simulink model "lots_of_connections"  (Simulink 7.6)
settings: Solver=FixedStepDiscrete  StartTime=0.0  StopTime=0  RelTol=1e-3
values from neighbouring files (symbols this model uses):
  Iter_Segment_Thresh = 60    [VisionConstants.m]
  Scale_Forward_B = 0    [VisionConstants.m]
  Scale_Forward_G = 1    [VisionConstants.m]
  Scale_Forward_H = 1    [VisionConstants.m]
  Scale_Forward_R = 0    [VisionConstants.m]
  Scale_Forward_S = 1    [VisionConstants.m]
  Scale_Forward_V = 5    [VisionConstants.m]
undefined symbols (not defined in the file or in its folder): black_al, black_au, black_bl, black_bu, blue_al, blue_au, blue_bl, blue_bu, gray, green_al, green_au, green_bl, green_bu, orange_al, orange_au, orange_bl, orange_bu, Rec, red_al, red_au, red_bl, red_bu, SDTV, yellow_al, yellow_au, yellow_bl, yellow_bu
libraries: vipconversions x4, vipgeotforms x3, vipsnks x2, vipsrcs x1
settings Model: Creator=Thing 1  LastModifiedBy=auvt
settings OptimizationCC: InlineParams=on  OptimizeModelRefInitCode=on
settings RTWCC: SystemTargetFile=ert.tlc  GenCodeOnly=on  TemplateMakefile=ert_default_tmf  Description=Real-Time Workshop Embedded Coder  GenerateReport=on  ProcessScript=ert_make_rtw_hook  IncludeHyperlinkInReport=on  LaunchReport=on  TargetLang=C++
settings CodeAppCC: IgnoreCustomStorageClasses=off
settings ERTTargetCC: MultiwordLength=2048  GenerateSampleERTMain=on  IncludeMdlTerminateFcn=off  ERTCustomFileTemplate=example_file_process.tlc  ConvertIfToSwitch=off

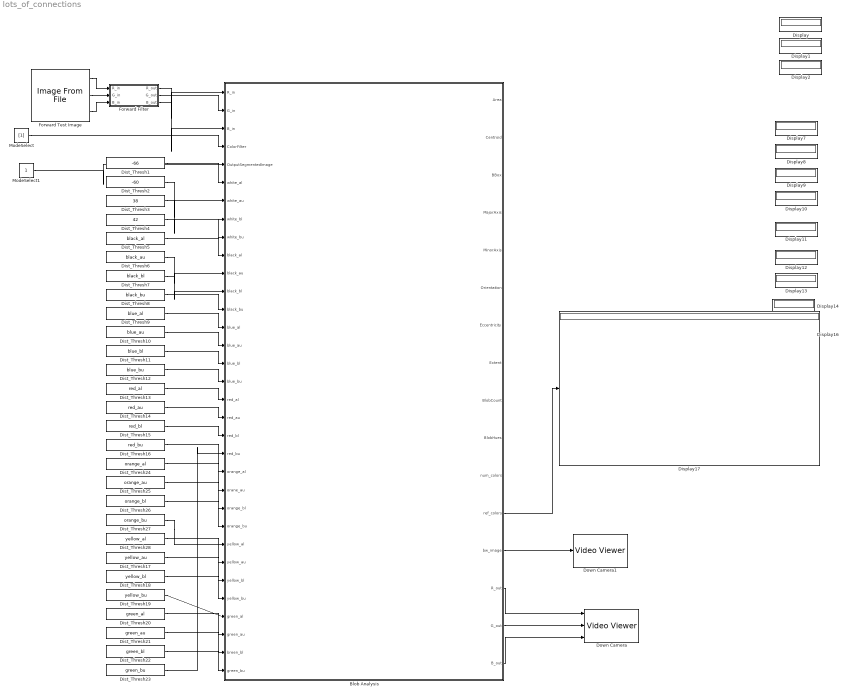
== system lots_of_connections ==
  Blob Analysis : Subsystem
  Display{,1..2,7..14,16..17} (13 alike) : Display
  Dist_Thresh1 : Constant  Value=-66  SampleTime=-1
  Dist_Thresh10 : Constant  Value=blue_au  SampleTime=-1
  Dist_Thresh11 : Constant  Value=blue_bl  SampleTime=-1
  Dist_Thresh12 : Constant  Value=blue_bu  SampleTime=-1
  Dist_Thresh13 : Constant  Value=red_al  SampleTime=-1
  Dist_Thresh14 : Constant  Value=red_au  SampleTime=-1
  Dist_Thresh15 : Constant  Value=red_bl  SampleTime=-1
  Dist_Thresh16 : Constant  Value=red_bu  SampleTime=-1
  Dist_Thresh17 : Constant  Value=yellow_au  SampleTime=-1
  Dist_Thresh18 : Constant  Value=yellow_bl  SampleTime=-1
  Dist_Thresh19 : Constant  Value=yellow_bu  SampleTime=-1
  Dist_Thresh2 : Constant  Value=-60  SampleTime=-1
  Dist_Thresh20 : Constant  Value=green_al  SampleTime=-1
  Dist_Thresh21 : Constant  Value=green_au  SampleTime=-1
  Dist_Thresh22 : Constant  Value=green_bl  SampleTime=-1
  Dist_Thresh23 : Constant  Value=green_bu  SampleTime=-1
  Dist_Thresh24 : Constant  Value=orange_al  SampleTime=-1
  Dist_Thresh25 : Constant  Value=orange_au  SampleTime=-1
  Dist_Thresh26 : Constant  Value=orange_bl  SampleTime=-1
  Dist_Thresh27 : Constant  Value=orange_bu  SampleTime=-1
  Dist_Thresh28 : Constant  Value=yellow_al  SampleTime=-1
  Dist_Thresh3 : Constant  Value=38  SampleTime=-1
  Dist_Thresh4 : Constant  Value=42  SampleTime=-1
  Dist_Thresh5 : Constant  Value=black_al  SampleTime=-1
  Dist_Thresh6 : Constant  Value=black_au  SampleTime=-1
  Dist_Thresh7 : Constant  Value=black_bl  SampleTime=-1
  Dist_Thresh8 : Constant  Value=black_bu  SampleTime=-1
  Dist_Thresh9 : Constant  Value=blue_al  SampleTime=-1
  Down Camera : vipsnks/Video Viewer  DialogControllerArgs=DataTag4  inputType=Obsolete7b  imagePorts=Separate color signals  useColorMap=off  colormapValue=gray(256)  specRange=off  minInputVal=0  maxInputVal=255  FigPos=[565 773 364 553]  AxisZoom=on  trueSizedOnce=off  OpenAtMdlStart=on
  Down Camera1 : vipsnks/Video Viewer  DialogControllerArgs=DataTag6  inputType=Obsolete7b  imagePorts=One multidimensional signal  useColorMap=off  colormapValue=gray(256)  specRange=off  minInputVal=0  maxInputVal=255  FigPos=[955 767 364 553]  AxisZoom=on  trueSizedOnce=off  OpenAtMdlStart=on
  Forward Filter : Subsystem
  Forward Test Image : vipsrcs/Image From File  Tag=vipblks_nd  DialogController=vipDDGCreate  DialogControllerArgs=DataTag7  SystemSampleTime=-1  FileName=/home/auvt/auvc/src/vision/Test_Images/gate10.bmp  imagePorts=Separate color signals  Ts=-1  ImageDataType=double  Signed=on  WordLength=16  sdImageDataType=uint(8)  FractionLengthMode=User-defined  FractionLength=15  OutPortLabels=R|G|B
  ModeSelect : Constant  Value=[1]  SampleTime=-1
  ModeSelect1 : Constant  SampleTime=-1
  wires:
  Dist_Thresh1/1 -> Blob Analysis/6(white_al)
  Dist_Thresh2/1 -> Blob Analysis/7(white_au)
  Dist_Thresh3/1 -> Blob Analysis/8(white_bl)
  Dist_Thresh4/1 -> Blob Analysis/9(white_bu)
  Dist_Thresh5/1 -> Blob Analysis/10(black_al)
  Dist_Thresh6/1 -> Blob Analysis/11(black_au)
  Dist_Thresh7/1 -> Blob Analysis/12(black_bl)
  Dist_Thresh8/1 -> Blob Analysis/13(black_bu)
  Dist_Thresh9/1 -> Blob Analysis/14(blue_al)
  Dist_Thresh10/1 -> Blob Analysis/15(blue_au)
  Dist_Thresh11/1 -> Blob Analysis/16(blue_bl)
  Dist_Thresh12/1 -> Blob Analysis/17(blue_bu)
  Dist_Thresh13/1 -> Blob Analysis/18(red_al)
  Dist_Thresh14/1 -> Blob Analysis/19(red_au)
  Dist_Thresh15/1 -> Blob Analysis/20(red_bl)
  Dist_Thresh16/1 -> Blob Analysis/22(orange_al)
  Dist_Thresh24/1 -> Blob Analysis/23(orane_au)
  Dist_Thresh25/1 -> Blob Analysis/24(orange_bl)
  Dist_Thresh26/1 -> Blob Analysis/25(orange_bu)
  Dist_Thresh27/1 -> Blob Analysis/26(yellow_al)
  Dist_Thresh28/1 -> Blob Analysis/27(yellow_au)
  Dist_Thresh17/1 -> Blob Analysis/28(yellow_bl)
  Dist_Thresh18/1 -> Blob Analysis/29(yellow_bu)
  Dist_Thresh19/1 -> Blob Analysis/30(green_al)
  Dist_Thresh20/1 -> Blob Analysis/31(green_au)
  Dist_Thresh21/1 -> Blob Analysis/32(breen_bl)
  Dist_Thresh22/1 -> Blob Analysis/33(green_bu)
  Dist_Thresh23/1 -> Blob Analysis/21(red_bu)
  Blob Analysis/14(R_out) -> Down Camera/1
  Blob Analysis/15(G_out) -> Down Camera/2
  Blob Analysis/16(B_out) -> Down Camera/3
  ModeSelect/1 -> Blob Analysis/4(ColorFilter)
  ModeSelect1/1 -> Blob Analysis/5(OutputSegmentedImage)
  Blob Analysis/13(bw_image) -> Down Camera1/1
  Blob Analysis/12(ref_colors) -> Display17/1
  Forward Test Image/1 -> Forward Filter/1(R_in)
  Forward Test Image/2 -> Forward Filter/2(G_in)
  Forward Test Image/3 -> Forward Filter/3(B_in)
  Forward Filter/1(R_out) -> Blob Analysis/1(R_in)
  Forward Filter/2(G_out) -> Blob Analysis/2(G_in)
  Forward Filter/3(B_out) -> Blob Analysis/3(B_in)

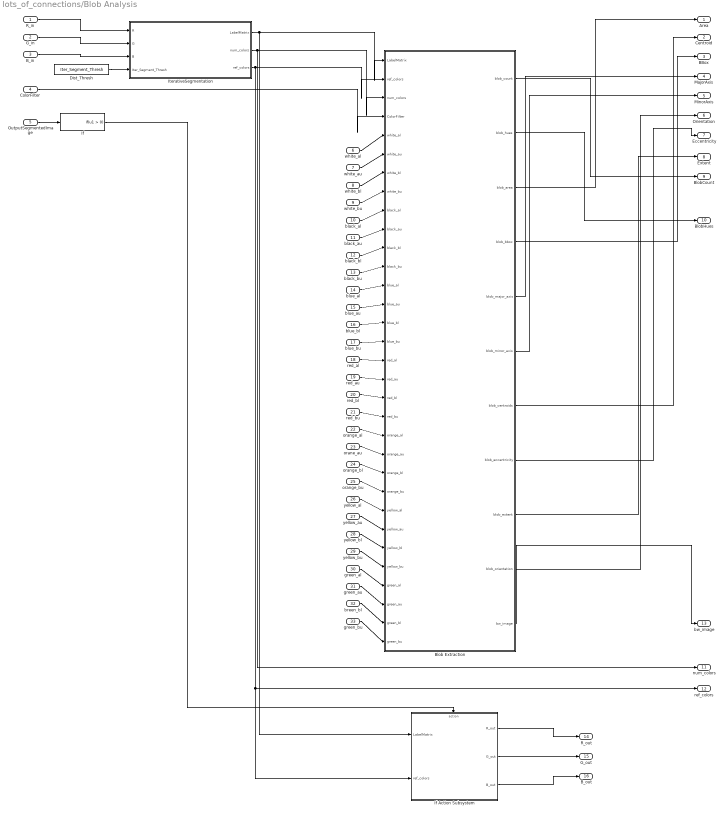
== system lots_of_connections/Blob Analysis ==
  R_in : Inport
  G_in : Inport  Port=2
  B_in : Inport  Port=3
  ColorFilter : Inport  Port=4
  OutputSegmentedImage : Inport  Port=5
  white_al : Inport  Port=6
  white_au : Inport  Port=7
  white_bl : Inport  Port=8
  white_bu : Inport  Port=9
  black_al : Inport  Port=10
  black_au : Inport  Port=11
  black_bl : Inport  Port=12
  black_bu : Inport  Port=13
  blue_al : Inport  Port=14
  blue_au : Inport  Port=15
  blue_bl : Inport  Port=16
  blue_bu : Inport  Port=17
  red_al : Inport  Port=18
  red_au : Inport  Port=19
  red_bl : Inport  Port=20
  red_bu : Inport  Port=21
  orange_al : Inport  Port=22
  orane_au : Inport  Port=23
  orange_bl : Inport  Port=24
  orange_bu : Inport  Port=25
  yellow_al : Inport  Port=26
  yellow_au : Inport  Port=27
  yellow_bl : Inport  Port=28
  yellow_bu : Inport  Port=29
  green_al : Inport  Port=30
  green_au : Inport  Port=31
  breen_bl : Inport  Port=32
  green_bu : Inport  Port=33
  Blob Extraction : Stateflow chart  TreatAsAtomicUnit=on
  Dist_Thresh : Constant  Value=Iter_Segment_Thresh  SampleTime=-1
  If : If  ShowElse=off
  If Action Subsystem : Subsystem  TreatAsAtomicUnit=on
  IterativeSegmentation : Subsystem
      settings: UndoDeleteFcn=Stateflow.SLINSF.SimulinkMan.restorePreDeleteFcn  PreDeleteFcn=Stateflow.SLINSF.SimulinkMan.removePreDeleteFcn
  Area : Outport
  Centroid : Outport  Port=2
  BBox : Outport  Port=3
  MajorAxis : Outport  Port=4
  MinorAxis : Outport  Port=5
  Orientation : Outport  Port=6
  Eccentricity : Outport  Port=7
  Extent : Outport  Port=8
  BlobCount : Outport  Port=9
  BlobHues : Outport  Port=10
  num_colors : Outport  Port=11
  ref_colors : Outport  Port=12
  bw_image : Outport  Port=13
  R_out : Outport  Port=14
  G_out : Outport  Port=15
  B_out : Outport  Port=16
  wires:
  IterativeSegmentation/1(LabelMatrix) -> Blob Extraction/1(LabelMatrix), If Action Subsystem/1(LabelMatrix)
  IterativeSegmentation/2(num_colors) -> Blob Extraction/3(num_colors), num_colors/1
  IterativeSegmentation/3(ref_colors) -> Blob Extraction/2(ref_colors), If Action Subsystem/2(ref_colors), ref_colors/1
  Blob Extraction/3(blob_area) -> Area/1
  Blob Extraction/7(blob_centroids) -> Centroid/1
  Blob Extraction/4(blob_bbox) -> BBox/1
  Blob Extraction/5(blob_major_axis) -> MajorAxis/1
  Blob Extraction/6(blob_minor_axis) -> MinorAxis/1
  Blob Extraction/10(blob_orientation) -> Orientation/1
  Blob Extraction/8(blob_eccentricity) -> Eccentricity/1
  Blob Extraction/9(blob_extent) -> Extent/1
  Blob Extraction/1(blob_count) -> BlobCount/1
  Blob Extraction/2(blob_hues) -> BlobHues/1
  ColorFilter/1 -> Blob Extraction/4(ColorFilter)
  Dist_Thresh/1 -> IterativeSegmentation/4(Iter_Segment_Thresh)
  R_in/1 -> IterativeSegmentation/1(R)
  G_in/1 -> IterativeSegmentation/2(G)
  B_in/1 -> IterativeSegmentation/3(B)
  white_al/1 -> Blob Extraction/5(white_al)
  white_au/1 -> Blob Extraction/6(white_au)
  white_bl/1 -> Blob Extraction/7(white_bl)
  white_bu/1 -> Blob Extraction/8(white_bu)
  black_al/1 -> Blob Extraction/9(black_al)
  black_au/1 -> Blob Extraction/10(black_au)
  black_bl/1 -> Blob Extraction/11(black_bl)
  black_bu/1 -> Blob Extraction/12(black_bu)
  blue_al/1 -> Blob Extraction/13(blue_al)
  blue_au/1 -> Blob Extraction/14(blue_au)
  blue_bl/1 -> Blob Extraction/15(blue_bl)
  blue_bu/1 -> Blob Extraction/16(blue_bu)
  red_al/1 -> Blob Extraction/17(red_al)
  red_au/1 -> Blob Extraction/18(red_au)
  red_bl/1 -> Blob Extraction/19(red_bl)
  red_bu/1 -> Blob Extraction/20(red_bu)
  orange_al/1 -> Blob Extraction/21(orange_al)
  orane_au/1 -> Blob Extraction/22(orange_au)
  orange_bl/1 -> Blob Extraction/23(orange_bl)
  orange_bu/1 -> Blob Extraction/24(orange_bu)
  yellow_al/1 -> Blob Extraction/25(yellow_al)
  yellow_au/1 -> Blob Extraction/26(yellow_au)
  yellow_bl/1 -> Blob Extraction/27(yellow_bl)
  yellow_bu/1 -> Blob Extraction/28(yellow_bu)
  green_al/1 -> Blob Extraction/29(green_al)
  green_au/1 -> Blob Extraction/30(green_au)
  breen_bl/1 -> Blob Extraction/31(green_bl)
  green_bu/1 -> Blob Extraction/32(green_bu)
  If/1 -> If Action Subsystem/Action
  OutputSegmentedImage/1 -> If/1
  If Action Subsystem/1(R_out) -> R_out/1
  If Action Subsystem/2(G_out) -> G_out/1
  If Action Subsystem/3(B_out) -> B_out/1
  Blob Extraction/11(bw_image) -> bw_image/1

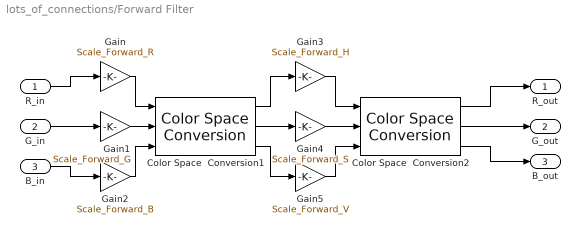
== system lots_of_connections/Forward Filter ==
  R_in : Inport  PortDimensions=Forward_Camera_Dimensions
  G_in : Inport  Port=2  PortDimensions=Forward_Camera_Dimensions
  B_in : Inport  Port=3  PortDimensions=Forward_Camera_Dimensions
  Color Space  Conversion1 : vipconversions/Color Space  Conversion  conversion=Obsolete  conversionActive=R'G'B' to HSV  wp_str=D50  rec=Rec. 601 (SDTV)  sys=1125/60/2:1  imagePorts=Separate color signals
  Color Space  Conversion2 : vipconversions/Color Space  Conversion  conversion=Obsolete  conversionActive=HSV to R'G'B'  wp_str=D50  rec=Rec. 601 (SDTV)  sys=1125/60/2:1  imagePorts=Separate color signals
  Gain : Gain  Gain=Scale_Forward_R
  Gain1 : Gain  Gain=Scale_Forward_G
  Gain2 : Gain  Gain=Scale_Forward_B
  Gain3 : Gain  Gain=Scale_Forward_H
  Gain4 : Gain  Gain=Scale_Forward_S
  Gain5 : Gain  Gain=Scale_Forward_V
  R_out : Outport  OutDataTypeStr=double
  G_out : Outport  Port=2  OutDataTypeStr=double
  B_out : Outport  Port=3  OutDataTypeStr=double
  wires:
  R_in/1 -> Gain/1
  G_in/1 -> Gain1/1
  B_in/1 -> Gain2/1
  Gain/1 -> Color Space  Conversion1/1
  Gain1/1 -> Color Space  Conversion1/2
  Gain2/1 -> Color Space  Conversion1/3
  Color Space  Conversion1/1 -> Gain3/1
  Color Space  Conversion1/2 -> Gain4/1
  Color Space  Conversion1/3 -> Gain5/1
  Gain3/1 -> Color Space  Conversion2/1
  Gain4/1 -> Color Space  Conversion2/2
  Gain5/1 -> Color Space  Conversion2/3
  Color Space  Conversion2/1 -> R_out/1
  Color Space  Conversion2/2 -> G_out/1
  Color Space  Conversion2/3 -> B_out/1

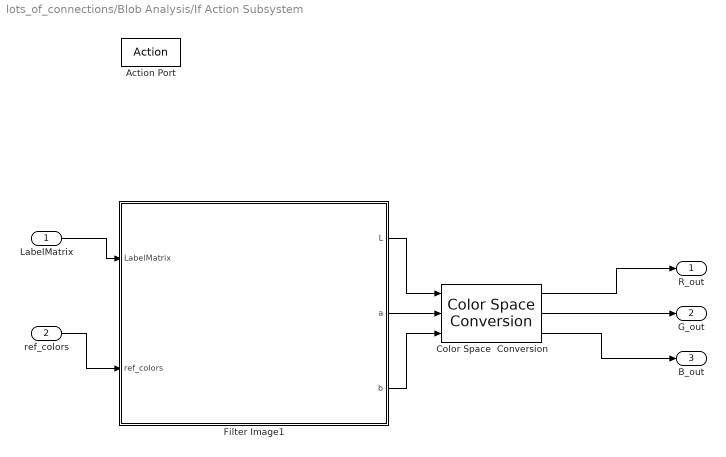
== system lots_of_connections/Blob Analysis/If Action Subsystem ==
  LabelMatrix : Inport
  ref_colors : Inport  Port=2
  Action Port : ActionPort  ActionType=then
  Color Space  Conversion : vipconversions/Color Space  Conversion  conversion=Obsolete  conversionActive=L*a*b* to sR'G'B'  wp_str=D65  rec=Rec. 601 (SDTV)  sys=1125/60/2:1  imagePorts=Separate color signals
  Filter Image1 : Stateflow chart  TreatAsAtomicUnit=on
  R_out : Outport
  G_out : Outport  Port=2
  B_out : Outport  Port=3
  wires:
  LabelMatrix/1 -> Filter Image1/1(LabelMatrix)
  ref_colors/1 -> Filter Image1/2(ref_colors)
  Filter Image1/1(L) -> Color Space  Conversion/1
  Filter Image1/2(a) -> Color Space  Conversion/2
  Filter Image1/3(b) -> Color Space  Conversion/3
  Color Space  Conversion/1 -> R_out/1
  Color Space  Conversion/2 -> G_out/1
  Color Space  Conversion/3 -> B_out/1

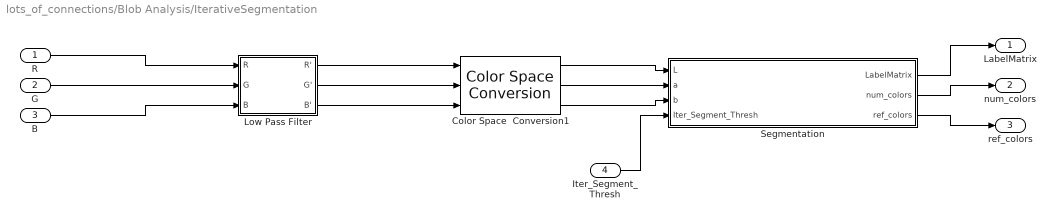
== system lots_of_connections/Blob Analysis/IterativeSegmentation ==
  R : Inport
  G : Inport  Port=2
  B : Inport  Port=3
  Iter_Segment_Thresh : Inport  Port=4
  Color Space  Conversion1 : vipconversions/Color Space  Conversion  conversion=Obsolete  conversionActive=sR'G'B' to L*a*b*  wp_str=D50  rec=Rec. 601 (SDTV)  sys=1125/60/2:1  imagePorts=Separate color signals
  Low Pass Filter : Subsystem
  Segmentation : Subsystem
  LabelMatrix : Outport
  num_colors : Outport  Port=2
  ref_colors : Outport  Port=3
  wires:
  Low Pass Filter/3(B') -> Color Space  Conversion1/3
  Low Pass Filter/2(G') -> Color Space  Conversion1/2
  Low Pass Filter/1(R') -> Color Space  Conversion1/1
  Color Space  Conversion1/3 -> Segmentation/3(b)
  Color Space  Conversion1/2 -> Segmentation/2(a)
  Color Space  Conversion1/1 -> Segmentation/1(L)
  R/1 -> Low Pass Filter/1(R)
  G/1 -> Low Pass Filter/2(G)
  B/1 -> Low Pass Filter/3(B)
  Segmentation/1(LabelMatrix) -> LabelMatrix/1
  Segmentation/2(num_colors) -> num_colors/1
  Segmentation/3(ref_colors) -> ref_colors/1
  Iter_Segment_Thresh/1 -> Segmentation/4(Iter_Segment_Thresh)

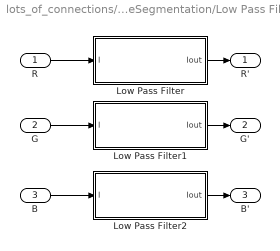
== system lots_of_connections/Blob Analysis/IterativeSegmentation/Low Pass Filter ==
  R : Inport
  G : Inport  Port=2
  B : Inport  Port=3
  Low Pass Filter : Stateflow chart  TreatAsAtomicUnit=on
  Low Pass Filter1 : Stateflow chart  TreatAsAtomicUnit=on
  Low Pass Filter2 : Stateflow chart  TreatAsAtomicUnit=on
  R' : Outport
  G' : Outport  Port=2
  B' : Outport  Port=3
  wires:
  Low Pass Filter/1(Iout) -> R'/1
  Low Pass Filter2/1(Iout) -> B'/1
  Low Pass Filter1/1(Iout) -> G'/1
  B/1 -> Low Pass Filter2/1(I)
  G/1 -> Low Pass Filter1/1(I)
  R/1 -> Low Pass Filter/1(I)

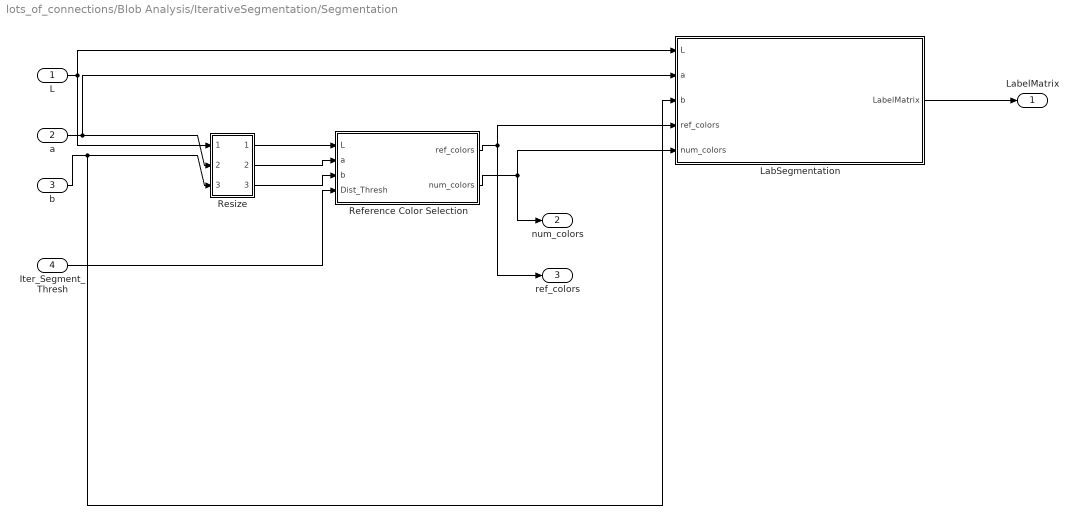
== system lots_of_connections/Blob Analysis/IterativeSegmentation/Segmentation ==
  L : Inport
  a : Inport  Port=2
  b : Inport  Port=3
  Iter_Segment_Thresh : Inport  Port=4
  LabSegmentation : Stateflow chart  TreatAsAtomicUnit=on
  Reference Color Selection : Stateflow chart  TreatAsAtomicUnit=on
  Resize : Subsystem
  LabelMatrix : Outport
  num_colors : Outport  Port=2
  ref_colors : Outport  Port=3
  wires:
  Iter_Segment_Thresh/1 -> Reference Color Selection/4(Dist_Thresh)
  LabSegmentation/1(LabelMatrix) -> LabelMatrix/1
  Reference Color Selection/2(num_colors) -> LabSegmentation/5(num_colors), num_colors/1
  Reference Color Selection/1(ref_colors) -> ref_colors/1, LabSegmentation/4(ref_colors)
  Resize/3(Out3) -> Reference Color Selection/3(b)
  Resize/2(Out2) -> Reference Color Selection/2(a)
  Resize/1(Out1) -> Reference Color Selection/1(L)
  b/1 -> LabSegmentation/3(b), Resize/3(In3)
  a/1 -> LabSegmentation/2(a), Resize/2(In2)
  L/1 -> LabSegmentation/1(L), Resize/1(In1)

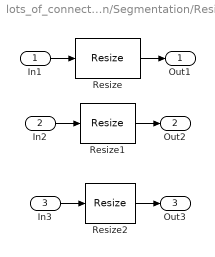
== system lots_of_connections/Blob Analysis/IterativeSegmentation/Segmentation/Resize ==
  In1 : Inport
  In2 : Inport  Port=2
  In3 : Inport  Port=3
  Resize : vipgeotforms/Resize  DialogController=vipDDGCreate  DialogControllerArgs=DataTag0  specify=Number of output rows and columns  rfactor=[]  outCols=25  outRows=25  outRowsCols=[60 80]  interp_method=Bilinear  antialias=on  useROI=off  roiFlag=off  prodOutputMode=Binary point scaling  prodOutputWordLength=32  prodOutputFracLength=10  roundingMode=Nearest  overflowMode=on
  Resize1 : vipgeotforms/Resize  DialogController=vipDDGCreate  DialogControllerArgs=DataTag1  specify=Number of output rows and columns  rfactor=[200 150]  outCols=25  outRows=25  outRowsCols=[60 80]  interp_method=Bilinear  antialias=on  useROI=off  roiFlag=off  prodOutputMode=Binary point scaling  prodOutputWordLength=32  prodOutputFracLength=10  roundingMode=Nearest  overflowMode=on
  Resize2 : vipgeotforms/Resize  DialogController=vipDDGCreate  DialogControllerArgs=DataTag2  specify=Number of output rows and columns  rfactor=[200 150]  outCols=25  outRows=25  outRowsCols=[60 80]  interp_method=Bilinear  antialias=on  useROI=off  roiFlag=off  prodOutputMode=Binary point scaling  prodOutputWordLength=32  prodOutputFracLength=10  roundingMode=Nearest  overflowMode=on
  Out1 : Outport
  Out2 : Outport  Port=2
  Out3 : Outport  Port=3
  wires:
  Resize2/1 -> Out3/1
  In3/1 -> Resize2/1
  Resize1/1 -> Out2/1
  In2/1 -> Resize1/1
  Resize/1 -> Out1/1
  In1/1 -> Resize/1

== matlab function Blob Analysis/Blob Extraction ==
  data: LabelMatrix input double; ref_colors input double; num_colors input double; blob_count output double; blob_hues output double; blob_area output double; blob_bbox output double; blob_major_axis output double; blob_minor_axis output double; blob_centroids output double; blob_eccentricity output double; blob_extent output double; blob_orientation output double; ColorFilter input double; bw_image output double; white_al input double; white_au input double; white_bl input double; white_bu input double; black_al input double; black_au input double; black_bl input double; black_bu input double; blue_al input double; blue_au input double; blue_bl input double; blue_bu input double; red_al input double; red_au input double; red_bl input double; red_bu input double; orange_al input double; orange_au input double; orange_bl input double; orange_bu input double; yellow_al input double; yellow_au input double; yellow_bl input double; yellow_bu input double; green_al input double; green_au input double; green_bl input double; green_bu input double
function [blob_count, blob_hues, blob_area, blob_bbox, blob_major_axis, blob_minor_axis, blob_centroids, blob_eccentricity, blob_extent, blob_orientation, bw_image] = GetBlobInfo(LabelMatrix, ref_colors, num_colors, ColorFilter,  white_al, white_au, white_bl, white_bu, black_al, black_au, black_bl, black_bu, blue_al, blue_au, blue_bl, blue_bu, red_al, red_au, red_bl, red_bu, orange_al, orange_au, orange_bl, orange_bu, yellow_al, yellow_au, yellow_bl, yellow_bu, green_al, green_au, green_bl, green_bu)



% This function calculates blob information for each color component after
%   iterative segmentation


% Initialize
max_num_blobs = 50;
min_blob_area = 5;

[rows, cols] = size(LabelMatrix);
LogicMatrix = false(rows,cols);
bw_image = zeros(rows,cols);

blob_count = 0;
blob_hues = zeros(3,max_num_blobs);

blob_area = -1.*ones(1,max_num_blobs);
blob_bbox = zeros(4,max_num_blobs);
blob_major_axis = zeros(1,max_num_blobs);
blob_minor_axis = zeros(1,max_num_blobs);
blob_centroids = zeros(2,max_num_blobs);
blob_eccentricity = zeros(1,max_num_blobs);
blob_extent = zeros(1,max_num_blobs);
blob_orientation = zeros(1,max_num_blobs);

max_num_col_filter = length(ColorFilter);
num_col_filter = max_num_col_filter;


% Populate a and b color component ranges for each color
a_range = zeros(2,max_num_col_filter);
b_range = zeros(2,max_num_col_filter);

c = 1;
for k = 1:max_num_col_filter
    if(ColorFilter(k) == 0)
        num_col_filter = k - 1;
        break;
    end
    
    switch(ColorFilter(k))
        case 1
            a_range(1,c) = white_al;
            a_range(2,c) = white_au;
            b_range(1,c) = white_bl;
            b_range(2,c) = white_bu;
        case 2
            a_range(1,c) = black_al;
            a_range(2,c) = black_au;
            b_range(1,c) = black_bl;
            b_range(2,c) = black_bu;
        case 3
            a_range(1,c) = blue_al;
            a_range(2,c) = blue_au;
            b_range(1,c) = blue_bl;
            b_range(2,c) = blue_bu;
        case 4
            a_range(1,c) = red_al;
            a_range(2,c) = red_au;
            b_range(1,c) = red_bl;
            b_range(2,c) = red_bu;
        case 5
            a_range(1,c) = orange_al;
            a_range(2,c) = orange_au;
            b_range(1,c) = orange_bl;
            b_range(2,c) = orange_bu;
        case 6
            a_range(1,c) = yellow_al;
            a_range(2,c) = yellow_au;
            b_range(1,c) = yellow_bl;
            b_range(2,c) = yellow_bu;
        case 7
            a_range(1,c) = green_al;
            a_range(2,c) = green_au;
            b_range(1,c) = green_bl;
            b_range(2,c) = green_bu;
    end
    
    c = c + 1;
    
end


% Input hblob, a matrix containing [Area, blob_centroids, Eccentricity] for each
% identified blob
persistent hblob
if isempty(hblob)
    hblob = video.BlobAnalysis('AreaOutputPort',true,'CentroidOutputPort',true,...
        'BoundingBoxOutputPort',true,'MajorAxisLengthOutputPort',true,'MinorAxisLengthOutputPort',true,...
        'OrientationOutputPort',true,...
        'EccentricityOutputPort',true,'ExtentOutputPort',true,'NumBlobsOutputPort',true,...
        'MinimumBlobAreaSource','Property','MinimumBlobArea', min_blob_area);
end


% Calculate geometric information about the blobs
%
% LogicMatrix is a binary version of LabelMatrix, with ones at all
%   locations for which color values are k, and zeros everywhere else
condition0 = (num_col_filter == 0);
for k = 1:num_colors
    
    condition1 = 0;
    
    if(condition0)
        condition1 = 1;
    else
        a = ref_colors(k, 2);
        b = ref_colors(k, 3);
        for i = 1:num_col_filter
            if( a >= a_range(1,i) && a <= a_range(2,i) && b >= b_range(1,i) && b <= b_range(2,i)  &&  (a_range(1,i)~=0 && a_range(2,i)~=0) )
                condition1 = 1;
                break;
            end
        end
    end
    
    if( condition1 == 1 )
        
        for i = 1:rows
            for j = 1:cols
                if(LabelMatrix(i,j) ~= k)
                    LogicMatrix(i,j) = false;
                else
                    LogicMatrix(i,j) = true;
                    bw_image(i,j) = 1;
                end
            end
        end

        [TArea,TCentroid,TBBox,TMajorAxis,TMinorAxis,TOrientation,TEccent,TExtent,TNumBlobs] = step(hblob,LogicMatrix);

        for i = 1:TNumBlobs
            if(blob_count + TNumBlobs <= max_num_blobs)

                blob_centroids(1,blob_count+i) = TCentroid(1,i);
                blob_centroids(2,blob_count+i) = TCentroid(2,i);

                ii = round(blob_centroids(1,blob_count+i));
                jj = round(blob_centroids(2,blob_count+i));

                blob_hues(1,blob_count+i) = ref_colors( LabelMatrix(ii,jj), 1 );
                blob_hues(2,blob_count+i) = ref_colors( LabelMatrix(ii,jj), 2 );
                blob_hues(3,blob_count+i) = ref_colors( LabelMatrix(ii,jj), 3 );

                blob_area(blob_count+i) = TArea(i);
                blob_bbox(blob_count+i) = TBBox(i);
                blob_major_axis(blob_count+i) = TMajorAxis(i);
                blob_minor_axis(blob_count+i) = TMinorAxis(i);
                blob_eccentricity(blob_count+i) = TEccent(i);
                blob_extent(blob_count+i) = TExtent(i);
                blob_orientation(blob_count+i) = TOrientation(i);

            end
        end

        blob_count = blob_count + double(TNumBlobs);

    end
    
end


return

== matlab function Blob Analysis/IterativeSegmentation/Low Pass Filter/Low Pass Filter2 ==
  data: I input double; Iout output double
function Iout = GaussianBlurr(I)
% This function calculates the gaussian blur of an intensity image

sigma = sqrt(2);

Grows = 3;    % Gaussian matrix rows
Gcols = 3;    % Gaussian matrix columns

[Irows Icols] = size(I);

Iout = double(zeros(Irows,Icols));

Trows = Irows - Grows + 1;
Tcols = Icols - Gcols + 1;
Itemp = double(zeros(Trows,Tcols));

G = zeros(Grows,Gcols);

FirstRow = ceil(-Grows/2);
LastRow = floor(Grows/2);
FirstCol = ceil(-Gcols/2);
LastCol = floor(Gcols/2);
Gsum = 0;
for i=FirstRow:LastRow
    for j = FirstCol:LastCol
        G(i-FirstRow+1,j-FirstCol+1) = exp(-(j*j+i*i)/(2*sigma*sigma));
        Gsum = Gsum + G(i-FirstRow+1,j-FirstCol+1);
    end
end

G = G./Gsum;

Itemp = conv2(double(I),double(G),'valid');

% reflect boundaries to keep image the same size
% top
Iout((1:LastRow),(LastCol+1:Icols-LastCol)) = Itemp((1:LastRow),(1:Tcols));
% bottom
Iout((Irows-LastRow+1:Irows),(LastCol+1:Icols-LastCol)) = Itemp((Trows-LastRow+1:Trows),(1:Tcols));
% left
Iout((1+LastRow:Irows-LastRow),(1:LastCol)) = Itemp((1:Trows),(1:LastCol));
% right
Iout((1+LastRow:Irows-LastRow),(Icols-LastCol+1:Icols)) = Itemp((1:Trows),(Tcols-LastCol+1:Tcols));
% center
Iout((1+LastRow:Irows-LastRow),(1+LastCol:Icols-LastCol)) = Itemp;
% top left corner
Iout(1:LastRow,1:LastCol) = Itemp(1:LastRow,1:LastCol);
% top right corner
Iout(1:LastRow,Icols-LastCol:Icols) = Itemp(1:LastRow,Tcols-LastCol:Tcols);
% bottom left corner
Iout(Irows-LastRow:Irows,1:LastCol) = Itemp(Trows-LastRow:Trows,1:LastCol);
% bottom right corner
Iout(Irows-LastRow:Irows,Icols-LastCol:Icols) = Itemp(Trows-LastRow:Trows,Tcols-LastCol:Tcols);

return

== matlab function Blob Analysis/If Action Subsystem/Filter Image1 ==
  data: LabelMatrix input double; ref_colors input double; L output double; a output double; b output double
function [L, a, b] = Display_Image(LabelMatrix, ref_colors)


% Initialize
[rows,cols] = size(LabelMatrix);
L = zeros(rows,cols);
a = zeros(rows,cols);
b = zeros(rows,cols);


% Allow only colors in specified range
for r = 1:rows
    for c = 1:cols
        
        L(r,c) = ref_colors(LabelMatrix(r,c), 1);
        a(r,c) = ref_colors(LabelMatrix(r,c), 2);
        b(r,c) = ref_colors(LabelMatrix(r,c), 3);
        
    end
end


return

== matlab function Blob Analysis/IterativeSegmentation/Low Pass Filter/Low Pass Filter ==
  data: I input double; Iout output double
function Iout = GaussianBlurr(I)
% This function calculates the gaussian blur of an intensity image

sigma = sqrt(2);

Grows = 3;    % Gaussian matrix rows
Gcols = 3;    % Gaussian matrix columns

[Irows Icols] = size(I);

Iout = double(zeros(Irows,Icols));

Trows = Irows - Grows + 1;
Tcols = Icols - Gcols + 1;
Itemp = double(zeros(Trows,Tcols));

G = zeros(Grows,Gcols);

FirstRow = ceil(-Grows/2);
LastRow = floor(Grows/2);
FirstCol = ceil(-Gcols/2);
LastCol = floor(Gcols/2);
Gsum = 0;
for i=FirstRow:LastRow
    for j = FirstCol:LastCol
        G(i-FirstRow+1,j-FirstCol+1) = exp(-(j*j+i*i)/(2*sigma*sigma));
        Gsum = Gsum + G(i-FirstRow+1,j-FirstCol+1);
    end
end

G = G./Gsum;

Itemp = conv2(double(I),double(G),'valid');

% reflect boundaries to keep image the same size
% top
Iout((1:LastRow),(LastCol+1:Icols-LastCol)) = Itemp((1:LastRow),(1:Tcols));
% bottom
Iout((Irows-LastRow+1:Irows),(LastCol+1:Icols-LastCol)) = Itemp((Trows-LastRow+1:Trows),(1:Tcols));
% left
Iout((1+LastRow:Irows-LastRow),(1:LastCol)) = Itemp((1:Trows),(1:LastCol));
% right
Iout((1+LastRow:Irows-LastRow),(Icols-LastCol+1:Icols)) = Itemp((1:Trows),(Tcols-LastCol+1:Tcols));
% center
Iout((1+LastRow:Irows-LastRow),(1+LastCol:Icols-LastCol)) = Itemp;
% top left corner
Iout(1:LastRow,1:LastCol) = Itemp(1:LastRow,1:LastCol);
% top right corner
Iout(1:LastRow,Icols-LastCol:Icols) = Itemp(1:LastRow,Tcols-LastCol:Tcols);
% bottom left corner
Iout(Irows-LastRow:Irows,1:LastCol) = Itemp(Trows-LastRow:Trows,1:LastCol);
% bottom right corner
Iout(Irows-LastRow:Irows,Icols-LastCol:Icols) = Itemp(Trows-LastRow:Trows,Tcols-LastCol:Tcols);

return

== matlab function Blob Analysis/IterativeSegmentation/Low Pass Filter/Low Pass Filter1 ==
  data: I input double; Iout output double
function Iout = GaussianBlurr(I)
% This function calculates the gaussian blur of an intensity image

sigma = sqrt(2);

Grows = 3;    % Gaussian matrix rows
Gcols = 3;    % Gaussian matrix columns

[Irows Icols] = size(I);

Iout = double(zeros(Irows,Icols));

Trows = Irows - Grows + 1;
Tcols = Icols - Gcols + 1;
Itemp = double(zeros(Trows,Tcols));

G = zeros(Grows,Gcols);

FirstRow = ceil(-Grows/2);
LastRow = floor(Grows/2);
FirstCol = ceil(-Gcols/2);
LastCol = floor(Gcols/2);
Gsum = 0;
for i=FirstRow:LastRow
    for j = FirstCol:LastCol
        G(i-FirstRow+1,j-FirstCol+1) = exp(-(j*j+i*i)/(2*sigma*sigma));
        Gsum = Gsum + G(i-FirstRow+1,j-FirstCol+1);
    end
end

G = G./Gsum;

Itemp = conv2(double(I),double(G),'valid');

% reflect boundaries to keep image the same size
% top
Iout((1:LastRow),(LastCol+1:Icols-LastCol)) = Itemp((1:LastRow),(1:Tcols));
% bottom
Iout((Irows-LastRow+1:Irows),(LastCol+1:Icols-LastCol)) = Itemp((Trows-LastRow+1:Trows),(1:Tcols));
% left
Iout((1+LastRow:Irows-LastRow),(1:LastCol)) = Itemp((1:Trows),(1:LastCol));
% right
Iout((1+LastRow:Irows-LastRow),(Icols-LastCol+1:Icols)) = Itemp((1:Trows),(Tcols-LastCol+1:Tcols));
% center
Iout((1+LastRow:Irows-LastRow),(1+LastCol:Icols-LastCol)) = Itemp;
% top left corner
Iout(1:LastRow,1:LastCol) = Itemp(1:LastRow,1:LastCol);
% top right corner
Iout(1:LastRow,Icols-LastCol:Icols) = Itemp(1:LastRow,Tcols-LastCol:Tcols);
% bottom left corner
Iout(Irows-LastRow:Irows,1:LastCol) = Itemp(Trows-LastRow:Trows,1:LastCol);
% bottom right corner
Iout(Irows-LastRow:Irows,Icols-LastCol:Icols) = Itemp(Trows-LastRow:Trows,Tcols-LastCol:Tcols);

return

== matlab function Blob Analysis/IterativeSegmentation/Segmentation/LabSegmentation ==
  data: L input double; LabelMatrix output double; a input double; b input double; ref_colors input double; num_colors input double
function LabelMatrix  = LabSegmentation(L,a,b,ref_colors,num_colors)
% This function generates the label matrix

[rows cols] = size(L);
LabelMatrix = zeros(rows,cols);

for i = 1:rows
    for j = 1:cols
        min_dist = 1000;
        index = 1;
        for k = 1:num_colors
            dist = sqrt((ref_colors(k,1) - L(i,j))^2 + (ref_colors(k,2) - a(i,j))^2 + (ref_colors(k,3) - b(i,j))^2);
            if(dist < min_dist)
                min_dist = double(dist);
                index = k;
            end
        end
        LabelMatrix(i,j) = index;
    end
end


return

== matlab function Blob Analysis/IterativeSegmentation/Segmentation/Reference Color Selection ==
  data: L input double; ref_colors output double; a input double; b input double; num_colors output double; Dist_Thresh input double
function [ref_colors, num_colors] = Segmentation(L,a,b,Dist_Thresh)
% This function tries segmentation by adding new reference colors everytime
% a pixel is found with a distance greater than a certain amount from
% every other reference color

[rows cols] = size(L);

Dist_Threshold = Dist_Thresh;% L = 0 to 100, a = -100 to 100, b = -100 to 100
                    % max dist = 300 -> 60/300 is 20%
x = 1;  % coefficients determining distance calculation
y = 1.5;
z = 1.5;

max_num_colors = 50;
ref_colors = zeros(max_num_colors,3);   % At most 50 different reference colors
LabelMatrix = zeros(rows,cols);
num_colors = 1;

center_row = floor(rows/2);
center_col = floor(cols/2);

% Define first reference color to be colr
ref_colors(1,:) = [L(center_row,center_col) a(center_row,center_col) b(center_row,center_col)];

flag = 0;
i = 1;
j = 1;
while(i <= rows)        % perform initial segmentation
    while(i <= rows && flag == 0)
        while(j <= cols && flag == 0)
            k = 1;
            min_dist = 1000;
            index = 1;
            while(k <= num_colors)
                dist = sqrt(x*(ref_colors(k,1) - L(i,j))^2 + y*(ref_colors(k,2) - a(i,j))^2 + z*(ref_colors(k,3) - b(i,j))^2);
                if(min_dist > dist)
                    min_dist = double(dist);
                    index = k;
                end
                k = k + 1;
            end
            if(j == 117)
                cow = 1;
            end
            if(min_dist > Dist_Threshold && num_colors < max_num_colors)
                ref_colors(num_colors+1,:) = [L(i,j) a(i,j) b(i,j)];
                num_colors = num_colors + 1;
                flag = 1;
                i = 0;
                j = 0;
            else
                LabelMatrix(i,j) = index;
            end
            j = j + 1;
        end
        j = 1;
        i = i + 1;
    end
    flag = 0;
end

% Go through image once more to get more accurate values for the different regions
ref_color_L_avg = zeros(50,1);
ref_color_a_avg = zeros(50,1);
ref_color_b_avg = zeros(50,1);
color_count = zeros(50,1);
for i = 1:rows
    for j = 1:cols
        index = LabelMatrix(i,j);
        ref_color_L_avg(index) = ref_color_L_avg(index) + L(i,j);
        ref_color_a_avg(index) = ref_color_a_avg(index) + a(i,j);
        ref_color_b_avg(index) = ref_color_b_avg(index) + b(i,j);
        color_count(index) = color_count(index) + 1;
    end
end
ref_color_L_avg = ref_color_L_avg ./ color_count;
ref_color_a_avg = ref_color_a_avg ./ color_count;
ref_color_b_avg = ref_color_b_avg ./ color_count;

for i = 1:num_colors
    ref_colors(i,1) = ref_color_L_avg(i);
    ref_colors(i,2) = ref_color_a_avg(i);
    ref_colors(i,3) = ref_color_b_avg(i);
end

return
